simulink model "ClosedLoopFedbackSimPI_v1"  (R2022b)
settings: Solver=FixedStepDiscrete  StartTime=0.0  StopTime=600  FixedStep=1  RelTol=1e-3  AbsTol=1e-5
undefined symbols (not defined in the file or in its folder): DiscIntNeverNeededParam
libraries: simulink x3
settings Model: Creator=maxdonelan  LastModifiedBy=patrick
settings SolverCC: AlgebraicLoopSolver=TrustRegion
settings DataIOCC: SaveState=on
settings DebuggingCC: UnconnectedInputMsg=warning  UnconnectedOutputMsg=warning  UnconnectedLineMsg=warning  SFMachineParentedDataDiag=warning
settings ModelReferenceCC: EnableRefExpFcnMdlSchedulingChecks=on
settings SFSimCC: CustomCodeUndefinedFunction=UseInterfaceOnly

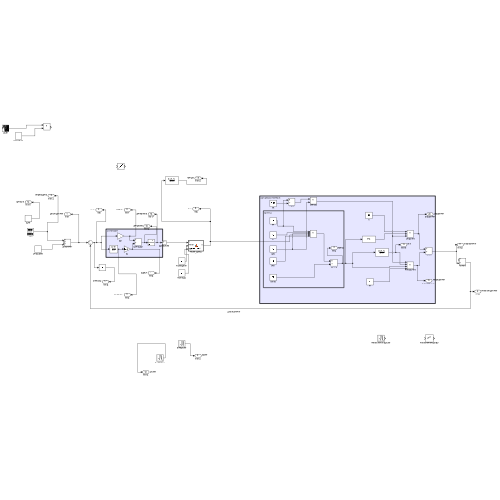
[thumbnail: Simulink's stored preview of the top-level diagram]
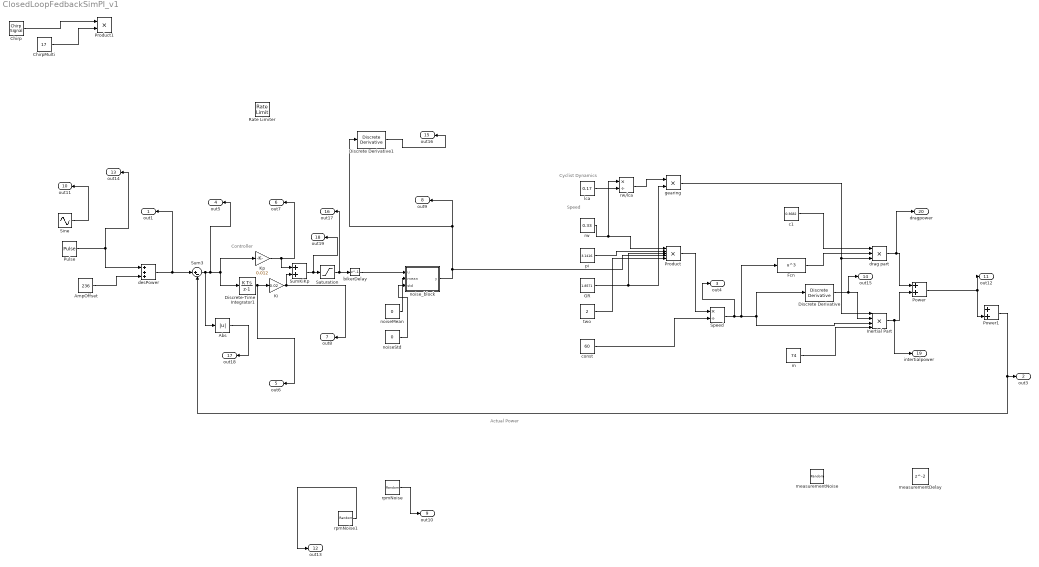
== system ClosedLoopFedbackSimPI_v1 ==
  note: Actual Power
  note: Controller
  note: Cyclist Dynamics
  note: Speed
  Abs : Abs  SaturateOnIntegerOverflow=off
  AmpOffset : Constant  Value=236
  Chirp : simulink/Sources/Chirp Signal  f1=0.0001  T=100  f2=0.01
  ChirpMulti : Constant  Value=17
  Discrete Derivative : simulink/Discrete/Discrete Derivative  gainval=1.0  ICPrevScaledInput=0.0  OutMin=[]  OutMax=[]  OutDataType=fixdt(1, 16)  OutScaling=2^-10  DoSatur=off
  Discrete Derivative1 : simulink/Discrete/Discrete Derivative  gainval=1.0  ICPrevScaledInput=0.0  OutMin=[]  OutMax=[]  OutDataType=fixdt(1, 16)  OutScaling=2^-10  DoSatur=off
  Discrete-Time Integrator1 : DiscreteIntegrator  SampleTime=-1  ICPrevOutput=DiscIntNeverNeededParam  ICPrevScaledInput=DiscIntNeverNeededParam
  Fcn : Fcn  Expr=u^3
  GR : Constant  Value=1.8571
  Inertial Part : Product  Inputs=4
  Ki : Gain  Gain=0.02
  Kp : Gain  Gain=0.012
  Power : Sum
  Power1 : Sum
  Product : Product  Inputs=5
  Product1 : Product
  Pulse : DiscretePulseGenerator  Amplitude=24  Period=1200  PulseWidth=600
  Rate Limiter : RateLimiter  RisingSlewLimit=100  FallingSlewLimit=-100
  Saturation : Saturate  UpperLimit=1000000  LowerLimit=0
  Sine : Sin  SineType=Sample based  Amplitude=100  Samples=20  SampleTime=600  Offset=10
  Speed : Product  Inputs=*/
  Sum3 : Sum  Inputs=|+-
  SumKiKp : Sum
  bikerDelay : Delay  DelayLength=1  InitialCondition=0
  c1 : Constant  Value=0.3682
  const : Constant  Value=60
  desPower : Sum  Inputs=+++
  drag part : Product  Inputs=3
  gearing : Product
  lca : Constant  Value=0.17
  m : Constant  Value=74
  measurementDelay : Delay  InitialCondition=0
  measurementNoise : RandomNumber  Variance=5  Seed=3  SampleTime=1
  noiseMean : Constant  Value=0
  noiseStd : Constant  Value=0
  noise_block : MATLAB Function  TreatAsAtomicUnit=on  SystemSampleTime=1
  pi : Constant  Value=3.1416
  rpmNoise : RandomNumber  Variance=2  Seed=2  SampleTime=1
  rpmNoise1 : RandomNumber  Variance=50  SampleTime=1
  rw : Constant  Value=0.33
  rw/lca : Product  Inputs=*/
  two : Constant  Value=2
  out1 : Outport  SignalName=desiredPower  VectorParamsAs1DForOutWhenUnconnected=off
  out3 : Outport  Port=2  SignalName=measuredPower  VectorParamsAs1DForOutWhenUnconnected=off
  out4 : Outport  Port=3  SignalName=speed  VectorParamsAs1DForOutWhenUnconnected=off
  out5 : Outport  Port=4  SignalName=error  VectorParamsAs1DForOutWhenUnconnected=off
  out6 : Outport  Port=5  SignalName=integrator  VectorParamsAs1DForOutWhenUnconnected=off
  out7 : Outport  Port=6  SignalName=Kpgain  VectorParamsAs1DForOutWhenUnconnected=off
  out8 : Outport  Port=7  SignalName=Kigain  VectorParamsAs1DForOutWhenUnconnected=off
  out9 : Outport  Port=8  SignalName=rpm  VectorParamsAs1DForOutWhenUnconnected=off
  out10 : Outport  Port=9  SignalName=Noise  VectorParamsAs1DForOutWhenUnconnected=off
  out11 : Outport  Port=10  SignalName=SineOut  VectorParamsAs1DForOutWhenUnconnected=off
  out12 : Outport  Port=11  SignalName=outputPower  VectorParamsAs1DForOutWhenUnconnected=off
  out13 : Outport  Port=12  SignalName=Noise1  VectorParamsAs1DForOutWhenUnconnected=off
  out14 : Outport  Port=13  SignalName=targetSignal  VectorParamsAs1DForOutWhenUnconnected=off
  out15 : Outport  Port=14  SignalName=acc  VectorParamsAs1DForOutWhenUnconnected=off
  out16 : Outport  Port=15  SignalName=rpmdot  VectorParamsAs1DForOutWhenUnconnected=off
  out17 : Outport  Port=16  SignalName=bpmaftersat  VectorParamsAs1DForOutWhenUnconnected=off
  out18 : Outport  Port=17  SignalName=threshold  VectorParamsAs1DForOutWhenUnconnected=off
  out19 : Outport  Port=18  SignalName=bpmbefsat  VectorParamsAs1DForOutWhenUnconnected=off
  intertialpower : Outport  Port=19  SignalName=inertialpower  VectorParamsAs1DForOutWhenUnconnected=off
  dragpower : Outport  Port=20  SignalName=dragpower  VectorParamsAs1DForOutWhenUnconnected=off
  wires:
  rw/1 -> Product/1, rw/lca/1
  pi/1 -> Product/2
  GR/1 -> gearing/2, Product/3
  Product/1 -> Speed/1
  const/1 -> Speed/2
  lca/1 -> rw/lca/2
  Speed/1 -> out4/1, Fcn/1, Discrete Derivative/1, Inertial Part/3
  rw/lca/1 -> gearing/1
  gearing/1 -> drag part/3, Inertial Part/1
  m/1 -> Inertial Part/4
  Fcn/1 -> drag part/2
  c1/1 -> drag part/1
  drag part/1 -> dragpower/1, Power/1
  Inertial Part/1 -> intertialpower/1, Power/2
  Sum3/1 -> Abs/1, out5/1, Kp/1, Discrete-Time Integrator1/1
  Discrete-Time Integrator1/1 -> out6/1, Ki/1
  Discrete Derivative/1 -> out15/1, Inertial Part/2
  Kp/1 -> out7/1, SumKiKp/1
  Ki/1 -> SumKiKp/2, out8/1
  noise_block/1(y) -> Product/4, out9/1, Discrete Derivative1/1
  desPower/1 -> out1/1, Sum3/1
  AmpOffset/1 -> desPower/3
  rpmNoise/1 -> out10/1
  Sine/1 -> out11/1
  Power/1 -> Power1/2, out12/1
  Power1/1 -> Sum3/2, out3/1
  rpmNoise1/1 -> out13/1
  Chirp/1 -> Product1/1
  ChirpMulti/1 -> Product1/2
  Pulse/1 -> desPower/1, out14/1
  Discrete Derivative1/1 -> out16/1
  Abs/1 -> out18/1
  two/1 -> Product/5
  noiseMean/1 -> noise_block/2(mean)
  noiseStd/1 -> noise_block/3(std)
  Saturation/1 -> bikerDelay/1, out17/1
  SumKiKp/1 -> out19/1, Saturation/1
  bikerDelay/1 -> noise_block/1(u)

== matlab function ClosedLoopFedbackSimPI_v1/noise_block ==
  data: u input; y output; mean input; std input
function y = noise_block(u, mean, std)
    if u > 0
        noise = std * randn;
        y = u + mean + noise;
    else
        y = 0;
    end
    
end
